simulink subsystem "IR_LED_Pattern"  (R2024b)
settings: Solver=VariableStepAuto  StartTime=0.0  StopTime=10.0  RelTol=1e-3
undefined symbols (not defined in the file or in its folder): IR_LED_PERIOD
settings Model: Creator=JesseJabezArendse  LastModifiedBy=JesseJabezArendse
settings RTWCC: GPUComputeCapability=3.5

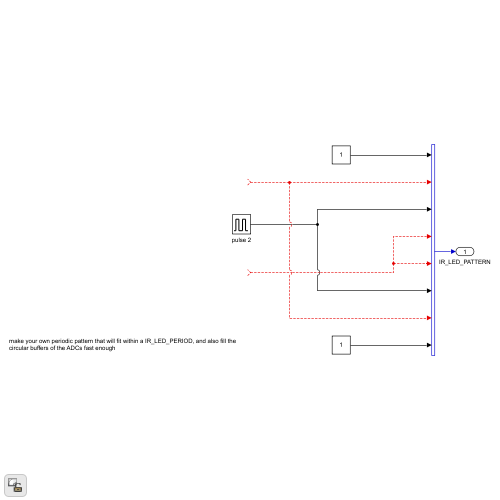
[thumbnail: Simulink's stored preview of the top-level diagram]
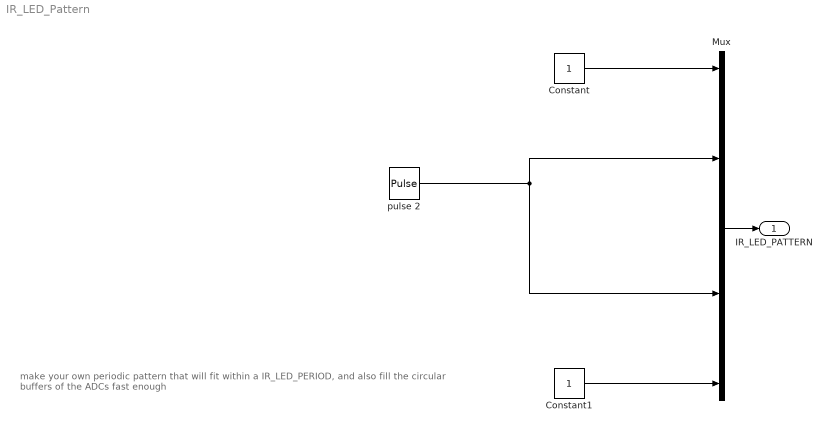
== system IR_LED_Pattern ==
  note: make your own periodic pattern that will fit within a IR_LED_PERIOD, and also fill the circular buffers of the ADCs fast enough
  Constant : Constant
  Constant1 : Constant
  Mux : Mux  Inputs=8
  pulse 2 : DiscretePulseGenerator  PulseType=Time based  Period=IR_LED_PERIOD  PulseWidth=1/4*100
  IR_LED_PATTERN : Outport
  wires:
  Constant/1 -> Mux/1
  Constant1/1 -> Mux/8
  ? -> Mux/7, Mux/2
  pulse 2/1 -> Mux/3, Mux/6
  ? -> Mux/5, Mux/4
  Mux/1 -> IR_LED_PATTERN/1
